simulink model "PMSM_2017b_1013"  (R2017b)
settings: Solver=FixedStepDiscrete  StartTime=0.0  StopTime=0.4  FixedStep=Ts  RelTol=1e-4  EnableMultiTasking=on
values from neighbouring files (symbols this model uses):
  AgSelector = 0    [initialization_1013.m]
  Ba = (Beta*J- Fl)/(1.5*P*flux)    [initialization_1013.m]
  Fl = 0.007*3/(100*pi)    (= 6.68450760986e-05)    [initialization_1013.m]
  flux = Kt/(1.5*P*sqrt(2))    [initialization_1013.m]
  fpwm = 1e4    (= 10000)    [initialization_1013.m]
  Imax = 6*sqrt(2)    [initialization_1013.m]
  J = 9.96e-5    (= 9.96e-05)    [initialization_1013.m]
  K1 = wn^2    (= 1000000)    [initialization_1013.m]
  K2 = 2*fei/wn    (= 0.003)    [initialization_1013.m]
  K_resolver = 1    [initialization_1013.m]
  Ki_Cctrl_d = Rs/(4*Tpwm)    (= 22125)    [initialization_1013.m]
  Ki_Cctrl_q = Rs/(4*Tpwm)    (= 22125)    [initialization_1013.m]
  Ki_Spdctrl = Beta*Kp_Spdctrl    [initialization_1013.m]
  Ki_Spdctrl_2 = 0.12*(pi*J)/(6000*P*flux*Tpwm^2)    [initialization_1013.m]
  Kp_Cctrl_d = Ld/(4*Tpwm)    (= 231.25)    [initialization_1013.m]
  Kp_Cctrl_q = Lq/(4*Tpwm)    (= 231.25)    [initialization_1013.m]
  Kp_Spdctrl = (Beta*J)/(1.5*P*flux)    [initialization_1013.m]
  Kp_Spdctrl_2 = 1*(pi*J)/(300*P*flux*Tpwm)    [initialization_1013.m]
  Kt = 1.32    [initialization_1013.m]
  Ld = Ls    (= 0.0925)    [initialization_1013.m]
  Lq = Ls    (= 0.0925)    [initialization_1013.m]
  Ls = 0.185/2    (= 0.0925)    [initialization_1013.m]
  P = 2    [initialization_1013.m]
  Rs = 17.7/2    (= 8.85)    [initialization_1013.m]
  SimMode = 1    [initialization_1013.m]
  TestCurrentController = 0    [initialization_1013.m]
  Tf = 0.08    [initialization_1013.m]
  Tpwm = 1e-4    (= 0.0001)    [initialization_1013.m]
  TqNorm = 0.6*9550/2500    (= 2.292)    [initialization_1013.m]
  Ts = 1e-6    (= 1e-06)    [initialization_1013.m]
  Udc = 230*sqrt(2)    [initialization_1013.m]
undefined symbols (not defined in the file or in its folder): A, B, DiscIntNeverNeededParam, f_LPF, f_LPF2, Init, K_SMO, Ki, Ki_PLL_SMO, Kp, Kp_PLL_SMO, LowerLimit, rate, UpperLimit
libraries: simulink x11, powerlib x7
(part 1 of 2)
settings Model: Creator=Joey Zhang  LastModifiedBy=Z0091619
settings SolverCC: ZeroCrossControl=DisableAll
settings DataIOCC: LimitDataPoints=on  SaveFormat=Array  SignalLoggingSaveFormat=ModelDataLogs
settings OptimizationCC: ExpressionDepthLimit=2147483647  InitFltsAndDblsToZero=on  LifeSpan=inf
settings DebuggingCC: UnderspecifiedInitializationDetection=Classic  MergeDetectMultiDrivingBlocksExec=none  SolverPrmCheckMsg=warning  FcnCallInpInsideContextMsg=warning  StateNameClashWarn=warning  SFUnexpectedBacktrackingDiag=warning  SFNoUnconditionalDefaultTransitionDiag=warning  SFExecutionAtInitializationDiag=none
settings HardwareCC: ProdBitPerPointer=32  ProdBitPerSizeT=32  ProdBitPerPtrDiffT=32  ProdLargestAtomicFloat=None  ProdIntDivRoundTo=Undefined  ProdEndianess=Unspecified  ProdWordSize=32  ProdHWDeviceType=32-bit Generic
settings ModelReferenceCC: PropagateSignalLabelsOutOfModel=off
settings CodeAppCC: StateflowObjectComments=on
settings GRTTargetCC: TargetLangStandard=C89/C90 (ANSI)  GeneratePreprocessorConditionals=Disable all  CombineOutputUpdateFcns=off  GRTInterface=on
settings ConfigComp: CovMetricSettings=dw  CovHtmlReporting=on  CovSaveCumulativeToWorkspaceVar=on  CovSaveSingleToWorkspaceVar=on  CovExternalEMLEnable=off
settings SimscapeCC: SimscapeNormalizeSystem=off

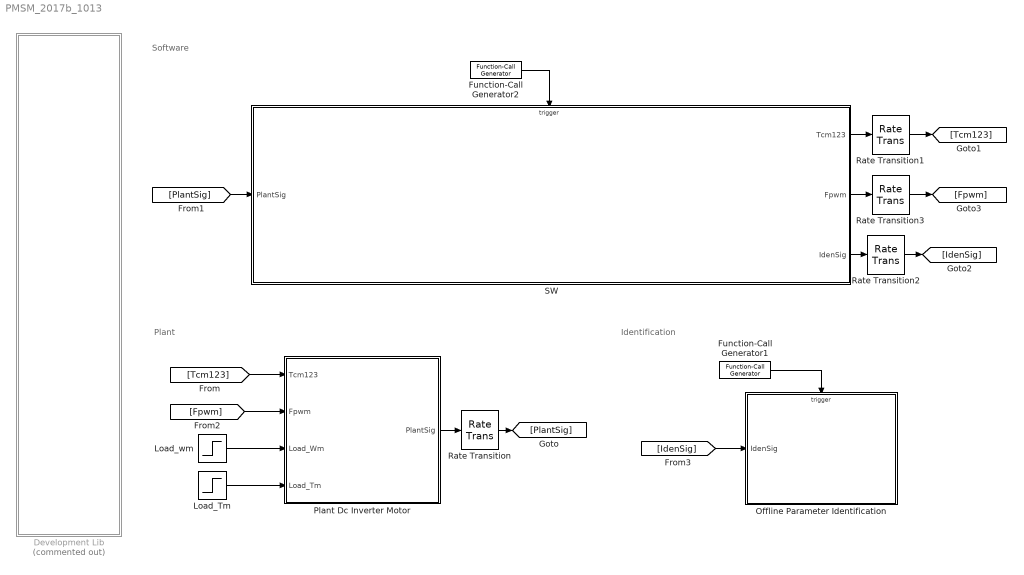
== system PMSM_2017b_1013 ==
  note: Software
  note: Plant
  note: Identification
  Development Lib : Subsystem  Commented=on
  Function-Call Generator1 : simulink/Ports & Subsystems/Function-Call Generator  sample_time=Tpwm  numberOfIterations=1
  Function-Call Generator2 : simulink/Ports & Subsystems/Function-Call Generator  sample_time=Tpwm  numberOfIterations=1
  Load_Tm : Step  After=TqNorm/2  SampleTime=0
  Load_wm : Step  Time=0.1  After=2500*pi/30  SampleTime=0
  Offline Parameter Identification : Subsystem
  Plant Dc Inverter Motor : Subsystem
  Rate Transition{,1..3} (4 alike) : RateTransition
  SW : Subsystem
  wires:
  Plant Dc Inverter Motor/1(PlantSig) -> Rate Transition/1
  SW/1(Tcm123) -> Rate Transition1/1
  SW/3(IdenSig) -> Rate Transition2/1
  [IdenSig] -> Offline Parameter Identification/1(IdenSig)
  Load_wm/1 -> Plant Dc Inverter Motor/3(Load_Wm)
  Load_Tm/1 -> Plant Dc Inverter Motor/4(Load_Tm)
  Function-Call Generator1/1 -> Offline Parameter Identification/Trigger
  Rate Transition/1 -> [PlantSig]
  [PlantSig] -> SW/1(PlantSig)
  [Tcm123] -> Plant Dc Inverter Motor/1(Tcm123)
  Rate Transition1/1 -> [Tcm123]
  Rate Transition2/1 -> [IdenSig]
  Function-Call Generator2/1 -> SW/Trigger
  SW/2(Fpwm) -> Rate Transition3/1
  Rate Transition3/1 -> [Fpwm]
  [Fpwm] -> Plant Dc Inverter Motor/2(Fpwm)

== system PMSM_2017b_1013/Development Lib ==
  AgRange(-pi,pi) : Subsystem
  Ag_atan2 : Subsystem
  Clamping_PI : Subsystem  Commented=on
  LPF1 : Subsystem
  Rate : Subsystem
  Speed : Subsystem  AncestorBlock=|  DialogController=POWERSYS.PowerSysDialog  mask(Discrete PI Controller){Kpw=Kp_Spdctrl, Kiw=Ki_Spdctrl, Ba=Ba, Par_Limits=[Imax -Imax], Init=0, Ts=-1}
      | powerlib_extras/Discrete 
      | Control Blocks/Discrete
      | PI Controller
      mask prompts: Kpw "Proportional gain (Kp):"; Kiw "Integral gain (Ki):"; Ba "feedback gain (Ba)"; Par_Limits "Output limits: [ Upper   Lower ]"; Init "Output initial value:"; Ts "Sample time:"
      mask help: This block implements a discrete PI controller.
      mask init:
      | UpperLimit=Par_Limits(1);
      | LowerLimit=Par_Limits(2);
      | power_initmask();
      mask Help: This block is part of a subset of blocks in the Extras library that does not have documentation associated with it, other than the block mask description.
      mask Display: disp('PI');
  TqEstimate : Subsystem  Commented=on
  UseMRASAg : Subsystem  Commented=on
  UseSMOAg : Subsystem  Commented=on
  pi-Id : Subsystem  AncestorBlock=|  DialogController=POWERSYS.PowerSysDialog  mask(Discrete PI Controller){Kp=Kp_Cctrl_d, Ki=Ki_Cctrl_d, Par_Limits=[Udc*sqrt(1/3) -Udc*sqrt(1/3)], Init=0, Ts=-1}
      | powerlib_extras/Discrete 
      | Control Blocks/Discrete
      | PI Controller
      mask prompts: Kp "Proportional gain (Kp):"; Ki "Integral gain (Ki):"; Par_Limits "Output limits: [ Upper   Lower ]"; Init "Output initial value:"; Ts "Sample time:"
      mask help: This block implements a discrete PI controller.
      mask init:
      | UpperLimit=Par_Limits(1);
      | LowerLimit=Par_Limits(2);
      | power_initmask();
      mask Help: This block is part of a subset of blocks in the Extras library that does not have documentation associated with it, other than the block mask description.
      mask Display: disp('PI');
  pi-Iq : Subsystem  AncestorBlock=|  DialogController=POWERSYS.PowerSysDialog  mask(Discrete PI Controller){Kp=Kp_Cctrl_q, Ki=Ki_Cctrl_q, Par_Limits=[Udc*sqrt(1/3) -Udc*sqrt(1/3)], Init=0, Ts=-1}
      | powerlib_extras/Discrete 
      | Control Blocks/Discrete
      | PI Controller
      mask prompts: Kp "Proportional gain (Kp):"; Ki "Integral gain (Ki):"; Par_Limits "Output limits: [ Upper   Lower ]"; Init "Output initial value:"; Ts "Sample time:"
      mask help: This block implements a discrete PI controller.
      mask init:
      | UpperLimit=Par_Limits(1);
      | LowerLimit=Par_Limits(2);
      | power_initmask();
      mask Help: This block is part of a subset of blocks in the Extras library that does not have documentation associated with it, other than the block mask description.
      mask Display: disp('PI');

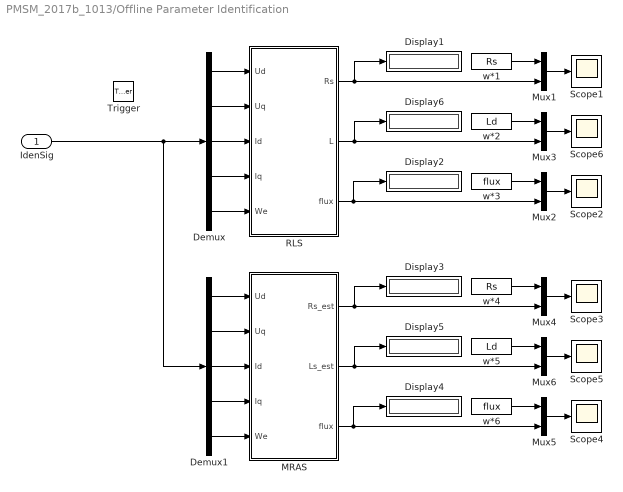
== system PMSM_2017b_1013/Offline Parameter Identification ==
  IdenSig : Inport
  Trigger : TriggerPort  TriggerType=function-call  VariantControl=Variant  PortDimensions=1
  Demux : Demux  Outputs=5
  Demux1 : Demux  Outputs=5
  Display{1..6} (6 alike) : Display
  MRAS : Subsystem
  Mux{1..6} (6 alike) : Mux  Inputs=2
  RLS : Subsystem
  Scope{1..6} (6 alike) : Scope
  w*1 : Constant  Value=Rs
  w*2 : Constant  Value=Ld
  w*3 : Constant  Value=flux
  w*4 : Constant  Value=Rs
  w*5 : Constant  Value=Ld
  w*6 : Constant  Value=flux
  wires:
  Mux3/1 -> Scope6/1
  RLS/2(L) -> Display6/1, Mux3/2
  w*2/1 -> Mux3/1
  w*1/1 -> Mux1/1
  RLS/1(Rs) -> Mux1/2, Display1/1
  Mux1/1 -> Scope1/1
  Mux2/1 -> Scope2/1
  RLS/3(flux) -> Display2/1, Mux2/2
  w*3/1 -> Mux2/1
  Demux/1 -> RLS/1(Ud)
  Demux/2 -> RLS/2(Uq)
  Demux/3 -> RLS/3(Id)
  Demux/4 -> RLS/4(Iq)
  Demux/5 -> RLS/5(We)
  Demux1/5 -> MRAS/5(We)
  Demux1/4 -> MRAS/4(Iq)
  Demux1/3 -> MRAS/3(Id)
  Demux1/2 -> MRAS/2(Uq)
  Demux1/1 -> MRAS/1(Ud)
  IdenSig/1 -> Demux1/1, Demux/1
  w*6/1 -> Mux5/1
  MRAS/3(flux) -> Mux5/2, Display4/1
  Mux5/1 -> Scope4/1
  Mux4/1 -> Scope3/1
  MRAS/1(Rs_est) -> Display3/1, Mux4/2
  w*4/1 -> Mux4/1
  w*5/1 -> Mux6/1
  MRAS/2(Ls_est) -> Mux6/2, Display5/1
  Mux6/1 -> Scope5/1

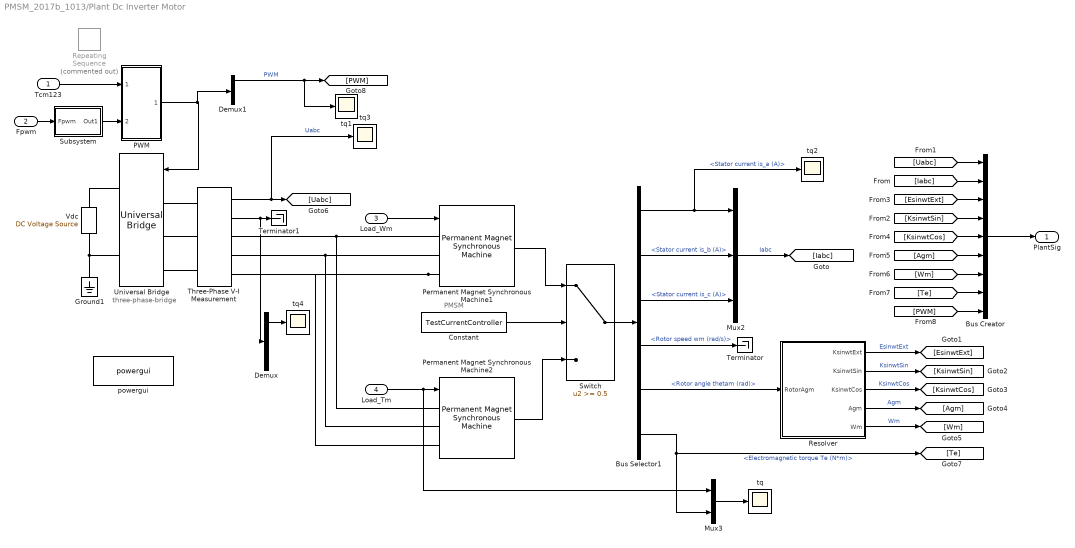
== system PMSM_2017b_1013/Plant Dc Inverter Motor ==
  note: three-phase-bridge
  note: PMSM
  Tcm123 : Inport
  Fpwm : Inport  Port=2
  Load_Wm : Inport  Port=3
  Load_Tm : Inport  Port=4
  Bus Creator : BusCreator  Inputs=9
  Bus Selector1 : BusSelector  OutputSignals=Stator current is_a (A),Stator current is_b (A),Stator current is_c (A),Rotor speed wm (rad/s),Rotor angle thetam (rad),Electromagnetic torque Te (N*m)
  Constant : Constant  Value=TestCurrentController
  Demux : Demux  Outputs=3
  Demux1 : Demux  Outputs=6
  Ground1 : powerlib/Elements/Ground  LConnTagsString=a
  Mux2 : Mux  Inputs=3
  Mux3 : Mux  Inputs=2
  PWM : Subsystem
  Permanent Magnet Synchronous Machine1 : powerlib/Machines/Permanent Magnet Synchronous Machine  NbPhases=3  FluxDistribution=Sinusoidal  RotorType=Round  MechanicalLoad=Speed w  PresetModel=No  ShowDetailedParameters=on  MeasurementBus=off  Resistance=Rs  Inductance=8.5e-3  dqInductances=[Ld Lq]  La=Ls  MachineConstant=Flux linkage established by magnets (V.s)  Flux=flux  VoltageCst=112.8644  TorqueCst=0.93338  Flat=120  Mechanical=[J Fl P Tf]  PolePairs=P  InitialConditions=[0,0,0,0]  InitialConditions5ph=[0 0 0 0 0 0]  TsPowergui=0  TsBlock=-1  RefAngle=Aligned with phase A axis (original Park)
      settings: SourceProductName=Simscape Power Systems
  Permanent Magnet Synchronous Machine2 : powerlib/Machines/Permanent Magnet Synchronous Machine  NbPhases=3  FluxDistribution=Sinusoidal  RotorType=Salient-pole  MechanicalLoad=Torque Tm  PresetModel=No  ShowDetailedParameters=on  MeasurementBus=off  Resistance=Rs  Inductance=8.5e-3  dqInductances=[Ld Lq]  La=Ls  MachineConstant=Flux linkage established by magnets (V.s)  Flux=flux  VoltageCst=112.8644  TorqueCst=0.93338  Flat=120  Mechanical=[J Fl P Tf]  PolePairs=P  InitialConditions=[0,0,0,0]  InitialConditions5ph=[0 0 0 0 0 0]  TsPowergui=0  TsBlock=-1  RefAngle=Aligned with phase A axis (original Park)
      settings: SourceProductName=Simscape Power Systems
  Repeating Sequence : simulink/Sources/Repeating Sequence  Commented=on  rep_seq_t=[0 Tpwm/2 Tpwm]  rep_seq_y=[0 Tpwm/2 0]
  Resolver : Subsystem
  Subsystem : Subsystem
  Switch : Switch  Threshold=0.5
  Terminator : Terminator
  Terminator1 : Terminator
  Three-Phase V-I Measurement : powerlib/Measurements/Three-Phase V-I Measurement  VoltageMeasurement=phase-to-ground  SetLabelV=off  LabelV=Vabc  Vpu=off  VpuLL=off  CurrentMeasurement=yes  SetLabelI=off  LabelI=Iabc  Ipu=off  Pbase=100e6  Vbase=500e3  OutputType=Complex  PhasorSimulation=off  PSBequivalent=0
  Universal Bridge : powerlib/Power Electronics/Universal Bridge  Arms=3  SnubberResistance=1e5  SnubberCapacitance=inf  Device=MOSFET / Diodes  Ron=1e-3  Lon=0  ForwardVoltages="[  0  0  ]"  ForwardVoltage=0  GTOparameters=[ 10e-6 , 20e-6 ]  IGBTparameters=[ 1e-6 , 2e-6 ]  Measurements=All voltages and currents  Measurements_2=None  converterType=Rectifier
  Vdc : powerlib/Electrical Sources/DC Voltage Source  Amplitude=Udc  Measurements=Voltage
  powergui : powerlib/powergui  SimulationMode=Discrete  SampleTime=Ts  frequency=60  Iterations=50  frequencyindice=0  Pbase=100e6  ErrMax=1e-4  UnitsV=kV  UnitsW=MW  buscounter=0  FunctionMessages=off  echomessages=off  EnableUseOfTLC=off  CurrentSourceSwitches=off  DisableSnubberDevices=off  DisableRonSwitches=off  DisableVfSwitches=off  DisplayEquations=off  SolverType=Backward Euler  Interpol=off  ExternalGateDelay=off  methode=off  Ts=0  x0status=blocks  SPID=off  SwTol=0  HookPort=off  RestoreLinks=warning  ResistiveCurrentMeasurement=off  Frange=[0:2:500]  Ylog=off  Xlog=on  ShowGrid=off  save=off  variable=ZData  structure=simout  ZoomFFT=off  StartTime=0.0  cycles=3  DisplayStyle=1  fundamental=60  FreqAxis=off  MaxFrequency=1000  frequencyindicesteady=1  RmsSteady=1  display=off
  tq{,1..4} (5 alike) : Scope
  PlantSig : Outport
  wires:
  Permanent Magnet Synchronous Machine1/1 -> Switch/1
  Switch/1 -> Bus Selector1/1
  Constant/1 -> Switch/2
  Mux3/1 -> tq/1
  Tcm123/1 -> PWM/1(Tcm123)
  Three-Phase V-I Measurement/1 -> tq3/1, [Uabc]  "Uabc"
  Mux2/1 -> [Iabc]  "Iabc"
  Permanent Magnet Synchronous Machine2/1 -> Switch/3
  Load_Tm/1 -> Mux3/1, Permanent Magnet Synchronous Machine2/1
  Bus Selector1/1 -> tq2/1, Mux2/1  "<Stator current is_a (A)>"
  Bus Selector1/2 -> Mux2/2  "<Stator current is_b (A)>"
  Bus Selector1/3 -> Mux2/3  "<Stator current is_c (A)>"
  Bus Selector1/5 -> Resolver/1(RotorAgm)  "<Rotor angle thetam (rad)>"
  Bus Selector1/4 -> Terminator/1  "<Rotor speed wm (rad/s)>"
  Three-Phase V-I Measurement/2 -> Demux/1, Terminator1/1
  Resolver/1(KsinwtExt) -> [EsinwtExt]  "EsinwtExt"
  Resolver/2(KsinwtSin) -> [KsinwtSin]  "KsinwtSin"
  Resolver/3(KsinwtCos) -> [KsinwtCos]  "KsinwtCos"
  Resolver/4(Agm) -> [Agm]  "Agm"
  Resolver/5(Wm) -> [Wm]  "Wm"
  Bus Selector1/6 -> [Te], Mux3/2  "<Electromagnetic torque Te (N*m)>"
  Bus Creator/1 -> PlantSig/1
  [Uabc] -> Bus Creator/1
  [Iabc] -> Bus Creator/2
  [EsinwtExt] -> Bus Creator/3
  [KsinwtSin] -> Bus Creator/4
  [KsinwtCos] -> Bus Creator/5
  [Agm] -> Bus Creator/6
  [Wm] -> Bus Creator/7
  [Te] -> Bus Creator/8
  Demux/1 -> tq4/1
  Load_Wm/1 -> Permanent Magnet Synchronous Machine1/1
  PWM/1(PWM) -> Demux1/1, Universal Bridge/1
  Demux1/1 -> tq1/1, [PWM]  "PWM"
  [PWM] -> Bus Creator/9
  Fpwm/1 -> Subsystem/1(Fpwm)
  Subsystem/1(Out1) -> PWM/2(Carrier)
  connections:
  Universal Bridge/RConn1 -- Vdc/RConn1
  Universal Bridge/RConn2 -- Ground1/LConn1 -- Vdc/LConn1
  Permanent Magnet Synchronous Machine1/LConn1 -- Three-Phase V-I Measurement/RConn1 -- Permanent Magnet Synchronous Machine2/LConn1
  Permanent Magnet Synchronous Machine1/LConn2 -- Three-Phase V-I Measurement/RConn2 -- Permanent Magnet Synchronous Machine2/LConn2
  Permanent Magnet Synchronous Machine1/LConn3 -- Permanent Magnet Synchronous Machine2/LConn3 -- Three-Phase V-I Measurement/RConn3
  Three-Phase V-I Measurement/LConn3 -- Universal Bridge/LConn3
  Universal Bridge/LConn2 -- Three-Phase V-I Measurement/LConn2
  Universal Bridge/LConn1 -- Three-Phase V-I Measurement/LConn1

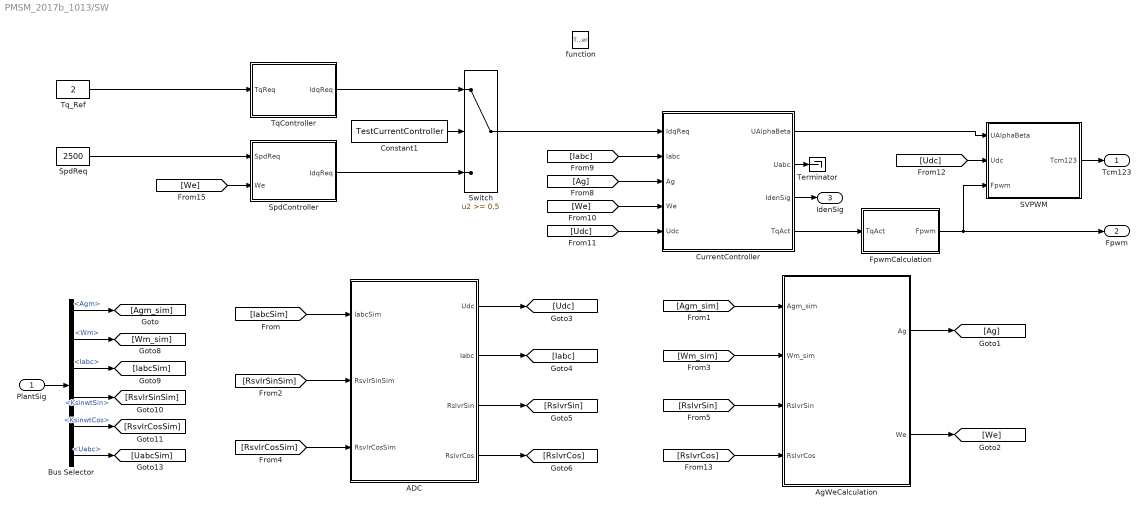
== system PMSM_2017b_1013/SW ==
  PlantSig : Inport
  function : TriggerPort  TriggerType=function-call  VariantControl=Variant
  ADC : Subsystem
  AgWeCalculation : Subsystem
  Bus Selector : BusSelector  OutputSignals=Agm,Wm,Iabc,KsinwtSin,KsinwtCos,Uabc
  Constant1 : Constant  Value=TestCurrentController
  CurrentController : Subsystem
  FpwmCalculation : Subsystem
  SVPWM : Subsystem
  SpdController : Subsystem
  SpdReq : Constant  Value=2500
  Switch : Switch  Threshold=0.5
  Terminator : Terminator
  TqController : Subsystem
  Tq_Ref : Constant  Value=2
  Tcm123 : Outport
  Fpwm : Outport  Port=2
  IdenSig : Outport  Port=3
  wires:
  Constant1/1 -> Switch/2
  SVPWM/1(Tcm123) -> Tcm123/1
  Tq_Ref/1 -> TqController/1(TqReq)
  TqController/1(IdqReq) -> Switch/1
  SpdReq/1 -> SpdController/1(SpdReq)
  SpdController/1(IdqReq) -> Switch/3
  Switch/1 -> CurrentController/1(IdqReq)
  CurrentController/1(UAlphaBeta) -> SVPWM/1(UAlphaBeta)
  AgWeCalculation/1(Ag) -> [Ag]
  AgWeCalculation/2(We) -> [We]
  [Ag] -> CurrentController/3(Ag)
  [Iabc] -> CurrentController/2(Iabc)
  [We] -> CurrentController/4(We)
  [Udc] -> CurrentController/5(Udc)
  [Udc] -> SVPWM/2(Udc)
  ADC/1(Udc) -> [Udc]
  ADC/2(Iabc) -> [Iabc]
  ADC/4(RslvrCos) -> [RslvrCos]
  ADC/3(RslvrSin) -> [RslvrSin]
  [Agm_sim] -> AgWeCalculation/1(Agm_sim)
  [Wm_sim] -> AgWeCalculation/2(Wm_sim)
  [RslvrSin] -> AgWeCalculation/3(RslvrSin)
  [RslvrCos] -> AgWeCalculation/4(RslvrCos)
  [We] -> SpdController/2(We)
  CurrentController/2(Uabc) -> Terminator/1
  PlantSig/1 -> Bus Selector/1
  Bus Selector/1 -> [Agm_sim]  "<Agm>"
  Bus Selector/2 -> [Wm_sim]  "<Wm>"
  Bus Selector/3 -> [IabcSim]  "<Iabc>"
  Bus Selector/4 -> [RsvlrSinSim]  "<KsinwtSin>"
  Bus Selector/5 -> [RsvlrCosSim]  "<KsinwtCos>"
  [IabcSim] -> ADC/1(IabcSim)
  [RsvlrCosSim] -> ADC/3(RsvlrCosSim)
  [RsvlrSinSim] -> ADC/2(RsvlrSinSim)
  Bus Selector/6 -> [UabcSim]  "<Uabc>"
  CurrentController/3(IdenSig) -> IdenSig/1
  CurrentController/4(TqAct) -> FpwmCalculation/1(TqAct)
  FpwmCalculation/1(Fpwm) -> Fpwm/1, SVPWM/3(Fpwm)

== system PMSM_2017b_1013/Development Lib/AgRange(-pi,pi) ==
  note: To make the Ag is in the range of [-pi,pi]
  Ag_RangeInf : Inport
  Constant : Constant  Value=pi
  Constant2 : Constant  Value=2*pi
  Mod : Math  Operator=mod  SaturateOnIntegerOverflow=on
  Relational Operator : RelationalOperator  OutDataTypeStr=boolean  RndMeth=Simplest
  Sum : Sum  Inputs=|+-
  Switch2 : Switch  Criteria=u2 > Threshold  Threshold=0.5
  Ag : Outport
  wires:
  Sum/1 -> Switch2/1
  Relational Operator/1 -> Switch2/2
  Ag_RangeInf/1 -> Mod/1
  Constant/1 -> Relational Operator/2
  Constant2/1 -> Sum/2, Mod/2
  Mod/1 -> Sum/1, Switch2/3, Relational Operator/1
  Switch2/1 -> Ag/1

== system PMSM_2017b_1013/Development Lib/Ag_atan2 ==
  Sin : Inport
  cos : Inport  Port=2
  Discrete Derivative : simulink/Discrete/Discrete Derivative  gainval=1.0  ICPrevScaledInput=0.0  OutMin=[]  OutMax=[]  OutDataType=fixdt(1, 16)  OutScaling=2^-10  DoSatur=off
  Sin1 : Trigonometry  Operator=atan2
  Ag : Outport
  we : Outport  Port=2
  wires:
  Sin/1 -> Sin1/1
  Sin1/1 -> Ag/1, Discrete Derivative/1
  Discrete Derivative/1 -> we/1
  cos/1 -> Sin1/2

== system PMSM_2017b_1013/Development Lib/Clamping_PI ==
  Error : Inport
  Udc : Inport  Port=2
  Abs : Abs
  Constant : Constant
  Constant1 : Constant  Value=0
  Discrete-Time Integrator : DiscreteIntegrator  IntegratorMethod=Integration: Trapezoidal  InitialCondition=Init  SampleTime=-1  UpperSaturationLimit=UpperLimit  LowerSaturationLimit=LowerLimit  ICPrevOutput=DiscIntNeverNeededParam  ICPrevScaledInput=DiscIntNeverNeededParam
  Gain : Gain  Gain=1/sqrt(3)
  Gain1 : Gain  Gain=-1
  Kp4 : Gain  Gain=Kp  SaturateOnIntegerOverflow=on  OutDataTypeStr=Inherit: Same as input  ParamDataTypeStr=Inherit: Same as input
  Kp5 : Gain  Gain=Ki  SaturateOnIntegerOverflow=on  OutDataTypeStr=Inherit: Same as input  ParamDataTypeStr=Inherit: Same as input
  Product : Product
  Relational Operator : RelationalOperator  OutDataTypeStr=boolean  RndMeth=Simplest
  Saturation Dynamic : simulink/Discontinuities/Saturation Dynamic  OutMin=[]  OutMax=[]  OutDataTypeStr=Inherit: Same as second input  OutDataType=fixdt(1, 16)  OutScaling=2^-10  DoSatur=off
  Sum6 : Sum  InputSameDT=on  OutDataTypeStr=Inherit: Same as first input
  Switch : Switch  Criteria=u2 > Threshold  Threshold=0.5
  Zero-Order Hold : ZeroOrderHold  SampleTime=-1
  Out : Outport  InitialOutput=0
  wires:
  Zero-Order Hold/1 -> Sum6/1
  Error/1 -> Kp5/1, Kp4/1
  Kp4/1 -> Zero-Order Hold/1
  Sum6/1 -> Saturation Dynamic/2, Abs/1
  Discrete-Time Integrator/1 -> Sum6/2
  Udc/1 -> Gain/1
  Gain/1 -> Saturation Dynamic/1, Relational Operator/1, Gain1/1
  Saturation Dynamic/1 -> Out/1
  Relational Operator/1 -> Switch/2
  Constant1/1 -> Switch/3
  Constant/1 -> Switch/1
  Switch/1 -> Product/2
  Kp5/1 -> Product/1
  Product/1 -> Discrete-Time Integrator/1
  Gain1/1 -> Saturation Dynamic/3
  Abs/1 -> Relational Operator/2

== system PMSM_2017b_1013/Development Lib/LPF1 ==
  u_in : Inport
  Add : Sum  Inputs=+-
  Add1 : Sum
  Constant : Constant  Value=Ts
  Constant1 : Constant  Value=f_LPF2
  Gain3 : Gain  Gain=2*pi
  Product : Product
  Product1 : Product
  Unit Delay : UnitDelay  SampleTime=-1
  u_out : Outport
  wires:
  Add1/1 -> Unit Delay/1, u_out/1
  Product/1 -> Product1/1
  Add/1 -> Product1/2
  Product1/1 -> Add1/1
  Gain3/1 -> Product/2
  Constant/1 -> Product/1
  Constant1/1 -> Gain3/1
  u_in/1 -> Add/1
  Unit Delay/1 -> Add/2, Add1/2

== system PMSM_2017b_1013/Development Lib/Rate ==
  In : Inport
  Abs : Abs
  Add : Sum  Inputs=+-
  Add1 : Sum
  Constant : Constant  Value=rate
  Product : Product
  Relational Operator : RelationalOperator  Operator=>  OutDataTypeStr=boolean  RndMeth=Simplest
  Switch1 : Switch  Criteria=u2 > Threshold
  Unit Delay : UnitDelay  SampleTime=-1
  Out1 : Outport
  wires:
  Relational Operator/1 -> Switch1/2
  Switch1/1 -> Out1/1
  In/1 -> Add1/1, Product/1, Switch1/3, Abs/1
  Unit Delay/1 -> Add/2
  Add/1 -> Relational Operator/1
  Constant/1 -> Product/2, Relational Operator/2
  Abs/1 -> Unit Delay/1, Add/1
  Add1/1 -> Switch1/1
  Product/1 -> Add1/2

== system PMSM_2017b_1013/Development Lib/Speed ==
  note: Discrete PID Controller
  Error : Inport
  Discrete-Time Integrator : DiscreteIntegrator  IntegratorMethod=Integration: Trapezoidal  InitialCondition=Init  SampleTime=-1  LimitOutput=on  UpperSaturationLimit=UpperLimit  LowerSaturationLimit=LowerLimit  ICPrevOutput=DiscIntNeverNeededParam  ICPrevScaledInput=DiscIntNeverNeededParam
  Kp1 : Gain  Gain=Ba  SaturateOnIntegerOverflow=on  OutDataTypeStr=Inherit: Same as input  ParamDataTypeStr=Inherit: Same as input
  Kp4 : Gain  Gain=Kpw  SaturateOnIntegerOverflow=on  OutDataTypeStr=Inherit: Same as input  ParamDataTypeStr=Inherit: Same as input
  Kp5 : Gain  Gain=Kiw  SaturateOnIntegerOverflow=on  OutDataTypeStr=Inherit: Same as input  ParamDataTypeStr=Inherit: Same as input
  Saturation2 : Saturate  UpperLimit=UpperLimit  LowerLimit=LowerLimit
  Scope : Scope
  Sum6 : Sum  Inputs=++-  SaturateOnIntegerOverflow=on  InputSameDT=on  OutDataTypeStr=Inherit: Same as first input
  Zero-Order Hold : ZeroOrderHold  SampleTime=-1
  Out : Outport  InitialOutput=0
  wires:
  Error/1 -> Kp4/1, Kp5/1
  Zero-Order Hold/1 -> Scope/1, Sum6/1
  Saturation2/1 -> Out/1
  Discrete-Time Integrator/1 -> Sum6/2
  Kp4/1 -> Zero-Order Hold/1
  Sum6/1 -> Saturation2/1
  Kp1/1 -> Sum6/3
  [Nr] -> Kp1/1
  Kp5/1 -> Discrete-Time Integrator/1

== system PMSM_2017b_1013/Development Lib/TqEstimate ==
  iq : Inport
  Gain : Gain  Gain=1.5*P*flux
  TqEst : Outport
  wires:
  Gain/1 -> TqEst/1
  iq/1 -> Gain/1

== system PMSM_2017b_1013/Development Lib/UseMRASAg ==
  note: 采用模型参考自适应算法估算电角度
  ud : Inport
  uq : Inport  Port=2
  id : Inport  Port=3
  iq : Inport  Port=4
  MRAS : Subsystem
  Ag_SMO : Outport
  We_SMO : Outport  Port=2

== system PMSM_2017b_1013/Development Lib/UseSMOAg ==
  note: 采用滑模控制 进行角度估算
  Uabc : Inport
  Iabc : Inport  Port=2
  Atan : Subsystem
  "PLL " : Subsystem
  Scope : Scope  NumInputPorts=2
  Scope1 : Scope  NumInputPorts=2
  Subsystem : Subsystem
  Ag_SMO : Outport
  We_SMO : Outport  Port=2
  wires:
  Iabc/1 -> Subsystem/2(Iabc)
  Uabc/1 -> Subsystem/1(Uabc)
  Subsystem/1(E_AlphaBeta) -> Atan/1(E_AlphaBeta), "PLL "/1(E_AlphaBeta)
  Atan/1(Ag_SMO) -> Scope/1
  Atan/2(we_SMO) -> Scope/2
  "PLL "/1(Ag_SMO) -> Ag_SMO/1, Scope1/1
  "PLL "/2(we_SMO) -> We_SMO/1, Scope1/2

== system PMSM_2017b_1013/Development Lib/pi-Id ==
  note: Discrete PID Controller
  Error : Inport  SampleTime=Ts
  Discrete-Time Integrator : DiscreteIntegrator  IntegratorMethod=Integration: Trapezoidal  InitialCondition=Init  SampleTime=-1  LimitOutput=on  UpperSaturationLimit=UpperLimit  LowerSaturationLimit=LowerLimit  ICPrevOutput=DiscIntNeverNeededParam  ICPrevScaledInput=DiscIntNeverNeededParam
  Kp4 : Gain  Gain=Kp  SaturateOnIntegerOverflow=on  OutDataTypeStr=Inherit: Same as input  ParamDataTypeStr=Inherit: Same as input
  Kp5 : Gain  Gain=Ki  SaturateOnIntegerOverflow=on  OutDataTypeStr=Inherit: Same as input  ParamDataTypeStr=Inherit: Same as input
  Saturation2 : Saturate  UpperLimit=UpperLimit  LowerLimit=LowerLimit
  Sum6 : Sum  SaturateOnIntegerOverflow=on  InputSameDT=on  OutDataTypeStr=Inherit: Same as first input
  Zero-Order Hold : ZeroOrderHold  SampleTime=-1
  Out : Outport  SampleTime=Ts  InitialOutput=0
  wires:
  Zero-Order Hold/1 -> Sum6/1
  Saturation2/1 -> Out/1
  Discrete-Time Integrator/1 -> Sum6/2
  Kp4/1 -> Zero-Order Hold/1
  Sum6/1 -> Saturation2/1
  Error/1 -> Kp5/1, Kp4/1
  Kp5/1 -> Discrete-Time Integrator/1

== system PMSM_2017b_1013/Development Lib/pi-Iq ==
  note: Discrete PID Controller
  Error : Inport  SampleTime=Ts
  Discrete-Time Integrator : DiscreteIntegrator  IntegratorMethod=Integration: Trapezoidal  InitialCondition=Init  SampleTime=-1  LimitOutput=on  UpperSaturationLimit=UpperLimit  LowerSaturationLimit=LowerLimit  ICPrevOutput=DiscIntNeverNeededParam  ICPrevScaledInput=DiscIntNeverNeededParam
  Kp4 : Gain  Gain=Kp  SaturateOnIntegerOverflow=on  OutDataTypeStr=Inherit: Same as input  ParamDataTypeStr=Inherit: Same as input
  Kp5 : Gain  Gain=Ki  SaturateOnIntegerOverflow=on  OutDataTypeStr=Inherit: Same as input  ParamDataTypeStr=Inherit: Same as input
  Saturation2 : Saturate  UpperLimit=UpperLimit  LowerLimit=LowerLimit
  Sum6 : Sum  SaturateOnIntegerOverflow=on  InputSameDT=on  OutDataTypeStr=Inherit: Same as first input
  Zero-Order Hold : ZeroOrderHold  SampleTime=-1
  Out : Outport  SampleTime=Ts  InitialOutput=0
  wires:
  Zero-Order Hold/1 -> Sum6/1
  Saturation2/1 -> Out/1
  Discrete-Time Integrator/1 -> Sum6/2
  Kp4/1 -> Zero-Order Hold/1
  Sum6/1 -> Saturation2/1
  Error/1 -> Kp5/1, Kp4/1
  Kp5/1 -> Discrete-Time Integrator/1

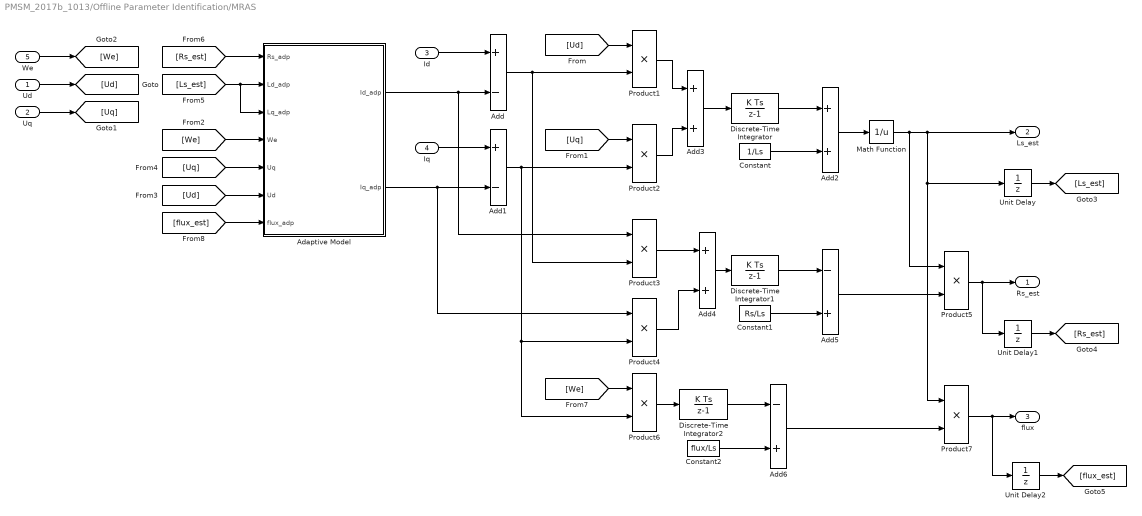
== system PMSM_2017b_1013/Offline Parameter Identification/MRAS ==
  Ud : Inport
  Uq : Inport  Port=2
  Id : Inport  Port=3
  Iq : Inport  Port=4
  We : Inport  Port=5
  Adaptive Model : Subsystem
  Add : Sum  Inputs=+-
  Add1 : Sum  Inputs=+-
  Add2 : Sum
  Add3 : Sum
  Add4 : Sum
  Add5 : Sum  Inputs=-+
  Add6 : Sum  Inputs=-+
  Constant : Constant  Value=1/Ls
  Constant1 : Constant  Value=Rs/Ls
  Constant2 : Constant  Value=flux/Ls
  Discrete-Time Integrator : DiscreteIntegrator  SampleTime=-1  UpperSaturationLimit=UpperLimit  LowerSaturationLimit=LowerLimit  ICPrevOutput=DiscIntNeverNeededParam  ICPrevScaledInput=DiscIntNeverNeededParam
  Discrete-Time Integrator1 : DiscreteIntegrator  SampleTime=-1  UpperSaturationLimit=UpperLimit  LowerSaturationLimit=LowerLimit  ICPrevOutput=DiscIntNeverNeededParam  ICPrevScaledInput=DiscIntNeverNeededParam
  Discrete-Time Integrator2 : DiscreteIntegrator  SampleTime=-1  UpperSaturationLimit=UpperLimit  LowerSaturationLimit=LowerLimit  ICPrevOutput=DiscIntNeverNeededParam  ICPrevScaledInput=DiscIntNeverNeededParam
  Math Function : Math  Operator=reciprocal  SaturateOnIntegerOverflow=on
  Product{1..7} (7 alike) : Product
  Unit Delay : UnitDelay  InitialCondition=Ls  SampleTime=-1
  Unit Delay1 : UnitDelay  InitialCondition=Rs  SampleTime=-1
  Unit Delay2 : UnitDelay  InitialCondition=flux  SampleTime=-1
  Rs_est : Outport
  Ls_est : Outport  Port=2
  flux : Outport  Port=3
  wires:
  Id/1 -> Add/1
  Iq/1 -> Add1/1
  Adaptive Model/2(Iq_adp) -> Product4/1, Add1/2
  Discrete-Time Integrator/1 -> Add2/1
  Ud/1 -> [Ud]
  [Ud] -> Product1/1
  We/1 -> [We]
  [Uq] -> Product2/1
  Add1/1 -> Product6/2, Product4/2, Product2/2
  Uq/1 -> [Uq]
  Product1/1 -> Add3/1
  Product2/1 -> Add3/2
  Add3/1 -> Discrete-Time Integrator/1
  Add2/1 -> Math Function/1
  Math Function/1 -> Product5/1, Product7/1, Unit Delay/1, Ls_est/1
  Constant/1 -> Add2/2
  [We] -> Adaptive Model/4(We)
  [Ud] -> Adaptive Model/6(Ud)
  [Uq] -> Adaptive Model/5(Uq)
  Adaptive Model/1(Id_adp) -> Product3/1, Add/2
  Add/1 -> Product3/2, Product1/2
  Product3/1 -> Add4/1
  Product4/1 -> Add4/2
  Constant1/1 -> Add5/2
  Discrete-Time Integrator1/1 -> Add5/1
  Add4/1 -> Discrete-Time Integrator1/1
  Add5/1 -> Product5/2
  Product5/1 -> Unit Delay1/1, Rs_est/1
  Unit Delay/1 -> [Ls_est]
  [Ls_est] -> Adaptive Model/3(Lq_adp), Adaptive Model/2(Ld_adp)
  Unit Delay1/1 -> [Rs_est]
  [Rs_est] -> Adaptive Model/1(Rs_adp)
  [We] -> Product6/1
  Product6/1 -> Discrete-Time Integrator2/1
  Constant2/1 -> Add6/2
  Discrete-Time Integrator2/1 -> Add6/1
  Add6/1 -> Product7/2
  Product7/1 -> Unit Delay2/1, flux/1
  Unit Delay2/1 -> [flux_est]
  [flux_est] -> Adaptive Model/7(flux_adp)

== system PMSM_2017b_1013/Offline Parameter Identification/RLS ==
  Ud : Inport
  Uq : Inport  Port=2
  Id : Inport  Port=3
  Iq : Inport  Port=4
  We : Inport  Port=5
  RLS : Subsystem
  RSL_1 : Subsystem
  Rs : Outport
  L : Outport  Port=2
  flux : Outport  Port=3
  wires:
  Ud/1 -> RLS/1(Ud), RSL_1/1(Ud)
  Uq/1 -> RLS/2(Uq), RSL_1/2(Uq)
  Iq/1 -> RLS/4(Iq), RSL_1/4(Iq)
  We/1 -> RLS/5(We), RSL_1/5(We)
  RSL_1/1(Rs) -> Rs/1
  RSL_1/2(L) -> L/1
  RSL_1/3(flux) -> flux/1
  Id/1 -> RLS/3(Id), RSL_1/3(Id)

== system PMSM_2017b_1013/Plant Dc Inverter Motor/PWM ==
  Tcm123 : Inport
  Carrier : Inport  Port=2
  Add : Sum  Inputs=+-
  Add1 : Sum  Inputs=+-
  Add2 : Sum  Inputs=+-
  Data Type Conversion : DataTypeConversion  OutDataTypeStr=double
  Data Type Conversion1 : DataTypeConversion  OutDataTypeStr=double
  Data Type Conversion2 : DataTypeConversion  OutDataTypeStr=double
  Demux : Demux  Outputs=3
  Logical Operator : Logic  Operator=NOT  AllPortsSameDT=off  OutDataTypeStr=boolean
  Logical Operator1 : Logic  Operator=NOT  AllPortsSameDT=off  OutDataTypeStr=boolean
  Logical Operator2 : Logic  Operator=NOT  AllPortsSameDT=off  OutDataTypeStr=boolean
  Mux : Mux  Inputs=6
  Mux1 : Mux  Inputs=2
  Relay : Relay  OffSwitchValue=-eps
  Relay1 : Relay  OffSwitchValue=-eps
  Relay2 : Relay  OffSwitchValue=-eps
  Te1 : Scope
  Te4 : Scope
  PWM : Outport
  wires:
  Demux/3 -> Add2/2
  Demux/2 -> Add1/2
  Demux/1 -> Te1/1, Mux1/2, Add/2
  Relay/1 -> Mux/5, Logical Operator2/1
  Relay1/1 -> Mux/3, Logical Operator1/1
  Mux/1 -> PWM/1
  Data Type Conversion/1 -> Mux/2
  Data Type Conversion1/1 -> Mux/4
  Data Type Conversion2/1 -> Mux/6
  Logical Operator2/1 -> Data Type Conversion2/1
  Logical Operator1/1 -> Data Type Conversion1/1
  Logical Operator/1 -> Data Type Conversion/1
  Add1/1 -> Relay1/1
  Add2/1 -> Relay/1
  Add/1 -> Relay2/1
  Tcm123/1 -> Demux/1
  Mux1/1 -> Te4/1
  Relay2/1 -> Mux/1, Logical Operator/1
  Carrier/1 -> Mux1/1, Add/1, Add2/1, Add1/1

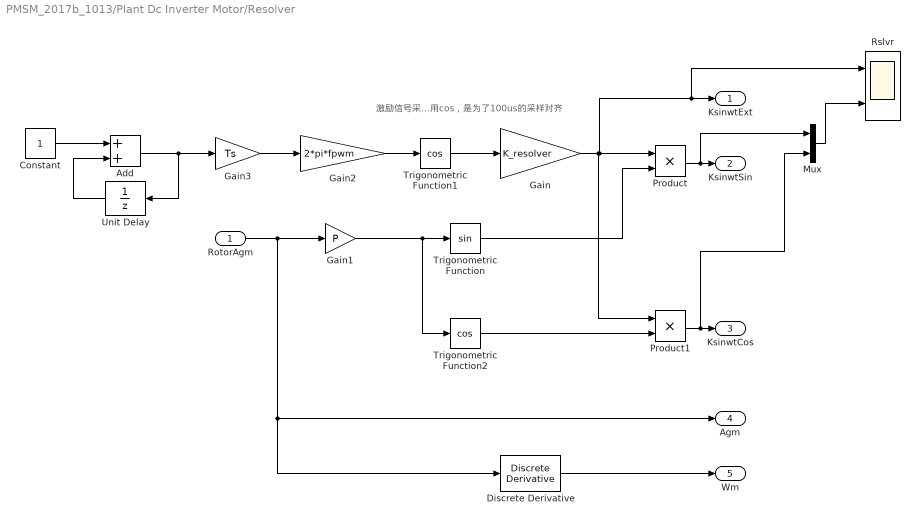
== system PMSM_2017b_1013/Plant Dc Inverter Motor/Resolver ==
  note: 激励信号采用cos，是为了100us的采样对齐
  RotorAgm : Inport
  Add : Sum
  Constant : Constant
  Discrete Derivative : simulink/Discrete/Discrete Derivative  gainval=1.0  ICPrevScaledInput=0.0  OutMin=[]  OutMax=[]  OutDataType=fixdt(1, 16)  OutScaling=2^-10  DoSatur=off
  Gain : Gain  Gain=K_resolver
  Gain1 : Gain  Gain=P
  Gain2 : Gain  Gain=2*pi*fpwm
  Gain3 : Gain  Gain=Ts
  Mux : Mux  Inputs=2
  Product : Product
  Product1 : Product
  Rslvr : Scope  NumInputPorts=2
  Trigonometric Function : Trigonometry
  Trigonometric Function1 : Trigonometry  Operator=cos
  Trigonometric Function2 : Trigonometry  Operator=cos
  Unit Delay : UnitDelay  SampleTime=-1
  KsinwtExt : Outport
  KsinwtSin : Outport  Port=2
  KsinwtCos : Outport  Port=3
  Agm : Outport  Port=4
  Wm : Outport  Port=5
  wires:
  Trigonometric Function1/1 -> Gain/1
  Gain2/1 -> Trigonometric Function1/1
  Gain/1 -> Rslvr/1, KsinwtExt/1, Product/1, Product1/1
  Trigonometric Function/1 -> Product/2
  Trigonometric Function2/1 -> Product1/2
  Product1/1 -> Mux/2, KsinwtCos/1
  Gain1/1 -> Trigonometric Function/1, Trigonometric Function2/1
  Discrete Derivative/1 -> Wm/1
  RotorAgm/1 -> Discrete Derivative/1, Agm/1, Gain1/1
  Product/1 -> Mux/1, KsinwtSin/1
  Mux/1 -> Rslvr/2
  Constant/1 -> Add/1
  Add/1 -> Gain3/1, Unit Delay/1
  Unit Delay/1 -> Add/2
  Gain3/1 -> Gain2/1

== system PMSM_2017b_1013/Plant Dc Inverter Motor/Subsystem ==
  Fpwm : Inport
  Add : Sum
  Add2 : Sum  Inputs=+-
  Constant1 : Constant
  Constant2 : Constant  Value=Ts
  Constant3 : Constant  Value=Ts
  Divide : Product  Inputs=*/
  Gain : Gain  Gain=0.5
  Math Function : Math  Operator=reciprocal  SaturateOnIntegerOverflow=on
  Mod : Math  Operator=mod  SaturateOnIntegerOverflow=on
  Product : Product
  Relational Operator : RelationalOperator  Operator=<  OutDataTypeStr=boolean  RndMeth=Simplest
  Switch1 : Switch  Criteria=u2 > Threshold  Threshold=0.5
  Te4 : Scope
  Unit Delay : UnitDelay  InitialCondition=-1  SampleTime=-1
  Out1 : Outport
  wires:
  Constant2/1 -> Divide/2
  Relational Operator/1 -> Switch1/2
  Gain/1 -> Relational Operator/2
  Unit Delay/1 -> Add/2
  Constant1/1 -> Add/1
  Fpwm/1 -> Math Function/1
  Switch1/1 -> Product/2, Te4/1
  Math Function/1 -> Divide/1
  Add/1 -> Unit Delay/1, Mod/1
  Divide/1 -> Gain/1, Mod/2, Add2/1
  Mod/1 -> Add2/2, Switch1/1, Relational Operator/1
  Add2/1 -> Switch1/3
  Product/1 -> Out1/1
  Constant3/1 -> Product/1

== system PMSM_2017b_1013/SW/ADC ==
  note: 实际DSP程序中，在此模块中进行 电流/电压/旋变的采样信号的标定 ，
      |
      | 默认是仿真模式
  IabcSim : Inport
  RsvlrSinSim : Inport  Port=2
  RsvlrCosSim : Inport  Port=3
  Constant{,1..3} (4 alike) : Constant  Value=SimMode
  IabcRaw : Constant
  RsvlrCosRaw : Constant
  RsvlrSinRaw : Constant
  Switch{,1..3} (4 alike) : Switch  Criteria=u2 > Threshold  Threshold=0.5
      settings: AttributesFormatString=%<Criteria>
  UdcRaw : Constant
  UdcSim : Constant  Value=Udc
  Udc : Outport
  Iabc : Outport  Port=2
  RslvrSin : Outport  Port=3
  RslvrCos : Outport  Port=4
  wires:
  Constant/1 -> Switch/2
  UdcSim/1 -> Switch/1
  UdcRaw/1 -> Switch/3
  Switch/1 -> Udc/1
  IabcSim/1 -> Switch1/1
  IabcRaw/1 -> Switch1/3
  Constant1/1 -> Switch1/2
  Switch1/1 -> Iabc/1
  Switch2/1 -> RslvrSin/1
  Constant2/1 -> Switch2/2
  Constant3/1 -> Switch3/2
  RsvlrSinSim/1 -> Switch2/1
  RsvlrSinRaw/1 -> Switch2/3
  RsvlrCosRaw/1 -> Switch3/3
  Switch3/1 -> RslvrCos/1
  RsvlrCosSim/1 -> Switch3/1

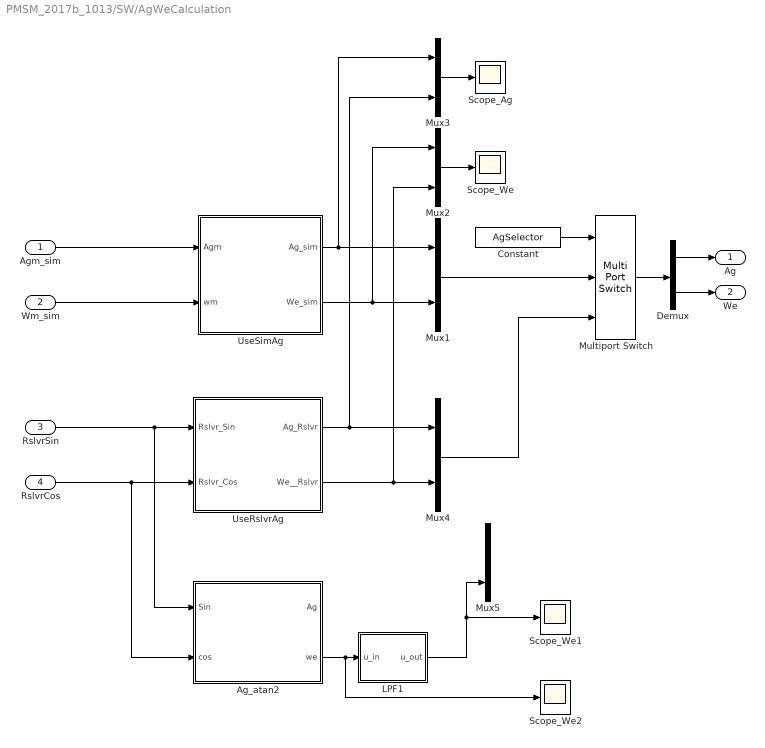
== system PMSM_2017b_1013/SW/AgWeCalculation ==
  Agm_sim : Inport
  Wm_sim : Inport  Port=2
  RslvrSin : Inport  Port=3
  RslvrCos : Inport  Port=4
  Ag_atan2 : Subsystem
  Constant : Constant  Value=AgSelector
  Demux : Demux  Outputs=2
  LPF1 : Subsystem
  Multiport Switch : MultiPortSwitch  DataPortOrder=Zero-based contiguous  Inputs=2
  Mux{1..5} (5 alike) : Mux  Inputs=2
  Scope_Ag : Scope
  Scope_We : Scope
  Scope_We1 : Scope
  Scope_We2 : Scope
  UseRslvrAg : Subsystem
  UseSimAg : Subsystem
  Ag : Outport
  We : Outport  Port=2
  wires:
  RslvrSin/1 -> Ag_atan2/1(Sin), UseRslvrAg/1(Rslvr_Sin)
  RslvrCos/1 -> Ag_atan2/2(cos), UseRslvrAg/2(Rslvr_Cos)
  Wm_sim/1 -> UseSimAg/2(wm)
  Agm_sim/1 -> UseSimAg/1(Agm)
  UseRslvrAg/1(Ag_Rslvr) -> Mux3/2, Mux4/1
  UseRslvrAg/2(We__Rslvr) -> Mux2/2, Mux4/2
  Mux1/1 -> Multiport Switch/2
  Constant/1 -> Multiport Switch/1
  Mux4/1 -> Multiport Switch/3
  Demux/1 -> Ag/1
  Demux/2 -> We/1
  UseSimAg/2(We_sim) -> Mux2/1, Mux1/2
  UseSimAg/1(Ag_sim) -> Mux3/1, Mux1/1
  Multiport Switch/1 -> Demux/1
  Mux3/1 -> Scope_Ag/1
  Mux2/1 -> Scope_We/1
  Ag_atan2/2(we) -> Scope_We2/1, LPF1/1(u_in)
  LPF1/1(u_out) -> Scope_We1/1, Mux5/2

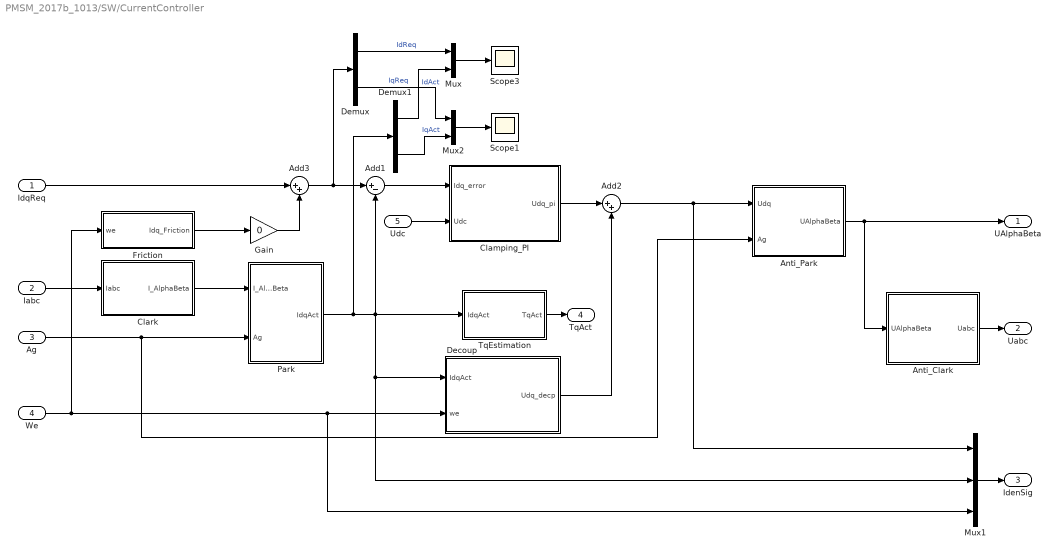
== system PMSM_2017b_1013/SW/CurrentController ==
  IdqReq : Inport
  Iabc : Inport  Port=2
  Ag : Inport  Port=3
  We : Inport  Port=4
  Udc : Inport  Port=5
  Add1 : Sum  Inputs=|+-
  Add2 : Sum  Inputs=|++
  Add3 : Sum  Inputs=|++
  Anti_Clark : Subsystem
  Anti_Park : Subsystem
  Clamping_PI : Subsystem
  Clark : Subsystem
  Decoup : Subsystem
  Demux : Demux  Outputs=2
  Demux1 : Demux  Outputs=2
  Friction : Subsystem
  Gain : Gain  Gain=0
  Mux : Mux  Inputs=2
  Mux1 : Mux  Inputs=3
  Mux2 : Mux  Inputs=2
  Park : Subsystem
  Scope1 : Scope
  Scope3 : Scope
  TqEstimation : Subsystem
  UAlphaBeta : Outport
  Uabc : Outport  Port=2
  IdenSig : Outport  Port=3
  TqAct : Outport  Port=4
  wires:
  We/1 -> Friction/1(we), Mux1/3, Decoup/2(we)
  Clark/1(I_AlphaBeta) -> Park/1(I_AlphaBeta)
  Iabc/1 -> Clark/1(Iabc)
  Ag/1 -> Anti_Park/2(Ag), Park/2(Ag)
  Anti_Park/1(UAlphaBeta) -> Anti_Clark/1(UAlphaBeta), UAlphaBeta/1
  Add1/1 -> Clamping_PI/1(Idq_error)
  Clamping_PI/1(Udq_pi) -> Add2/1
  Decoup/1(Udq_decp) -> Add2/2
  Udc/1 -> Clamping_PI/2(Udc)
  Anti_Clark/1(Uabc) -> Uabc/1
  Add2/1 -> Mux1/1, Anti_Park/1(Udq)
  Mux1/1 -> IdenSig/1
  Friction/1(Idq_Friction) -> Gain/1
  IdqReq/1 -> Add3/1
  Add3/1 -> Demux/1, Add1/1
  Gain/1 -> Add3/2
  Park/1(IdqAct) -> Demux1/1, TqEstimation/1(IdqAct), Mux1/2, Decoup/1(IdqAct), Add1/2
  Demux/1 -> Mux/1  "IdReq"
  Demux1/1 -> Mux/2  "IdAct"
  Mux2/1 -> Scope1/1
  Mux/1 -> Scope3/1
  Demux/2 -> Mux2/1  "IqReq"
  Demux1/2 -> Mux2/2  "IqAct"
  TqEstimation/1(TqAct) -> TqAct/1

== system PMSM_2017b_1013/SW/FpwmCalculation ==
  TqAct : Inport
  2-D Lookup Table : Lookup_n-D  NumberOfTableDimensions=1  BreakpointsForDimension1="[1  2  3  4]"  BreakpointsForDimension2=[1:3]  Table=[4000 6000 8000 10000]  InterpMethod=Flat  ExtrapMethod=Clip  InternalRulePriority=Speed  RndMeth=Simplest  InputSameDT=on
  Constant : Constant
  Constant1 : Constant  Value=10000
  Scope2 : Scope
  Switch : Switch  Criteria=u2 > Threshold  Threshold=0.5
  Fpwm : Outport
  wires:
  2-D Lookup Table/1 -> Switch/1
  TqAct/1 -> 2-D Lookup Table/1
  Switch/1 -> Scope2/1, Fpwm/1
  Constant/1 -> Switch/2
  Constant1/1 -> Switch/3

== system PMSM_2017b_1013/SW/SVPWM ==
  UAlphaBeta : Inport
  Udc : Inport  Port=2
  Fpwm : Inport  Port=3
  Demux : Demux  Outputs=2
  Math Function : Math  Operator=reciprocal  SaturateOnIntegerOverflow=on
  Sector Caculate : Subsystem
  T1T1 Caculate : Subsystem
  Tcm Caculate : Subsystem
  XYZ Caculate : Subsystem
  Tcm123 : Outport
  wires:
  Demux/2 -> Sector Caculate/2(Ubeta), XYZ Caculate/2(Ubeta)
  T1T1 Caculate/1(T1) -> Tcm Caculate/2(T1)
  Demux/1 -> Sector Caculate/1(Ualpha), XYZ Caculate/1(Ualpha)
  T1T1 Caculate/2(T2) -> Tcm Caculate/3(T2)
  Sector Caculate/1("N ") -> Tcm Caculate/1(N), T1T1 Caculate/1(N)
  XYZ Caculate/1(XYZ) -> T1T1 Caculate/2(XYZ)
  Math Function/1 -> XYZ Caculate/3(Tpwm), Tcm Caculate/4(Tpwm), T1T1 Caculate/3(Tpwm)
  Udc/1 -> XYZ Caculate/4(Udc)
  Tcm Caculate/1(Tcm1 Tcm2 Tcm3) -> Tcm123/1
  UAlphaBeta/1 -> Demux/1
  Fpwm/1 -> Math Function/1

== system PMSM_2017b_1013/SW/SpdController ==
  SpdReq : Inport
  We : Inport  Port=2
  Abs : Abs
  Add : Sum
  Add3 : Sum  Inputs=|+-
  Clamping_PI : Subsystem
  Clamping_PI1 : Subsystem  Commented=on
  Constant : Constant
  Discrete-Time Integrator : DiscreteIntegrator  SampleTime=-1  UpperSaturationLimit=UpperLimit  LowerSaturationLimit=LowerLimit  ICPrevOutput=DiscIntNeverNeededParam  ICPrevScaledInput=DiscIntNeverNeededParam
  EOT : Subsystem
  Gain : Gain  Gain=Tpwm
  Mux5 : Mux  Inputs=2
  Product : Product
  Scope1 : Scope
  Scope2 : Scope
  Scope3 : Scope
  Unit Delay : UnitDelay  SampleTime=-1
  we2wm : Gain  Gain=1/P
  wm2Nr : Gain  Gain=30/pi
  IdqReq : Outport
  wires:
  Mux5/1 -> Scope1/1
  we2wm/1 -> wm2Nr/1
  wm2Nr/1 -> Clamping_PI/2(SpdAct), Add3/2, Mux5/2  "SpdAct"
  EOT/1(IdqReq) -> IdqReq/1
  SpdReq/1 -> Mux5/1, Add3/1
  We/1 -> we2wm/1
  Add3/1 -> Abs/1, Clamping_PI1/1(Spd_error), Clamping_PI/1(Spd_error)
  Clamping_PI1/1(IqReq) -> Scope2/1
  Abs/1 -> Product/1
  Constant/1 -> Add/1
  Add/1 -> Gain/1, Unit Delay/1
  Unit Delay/1 -> Add/2
  Gain/1 -> Product/2
  Product/1 -> Discrete-Time Integrator/1
  Discrete-Time Integrator/1 -> Scope3/1  "ITAE"
  Clamping_PI/1(IqReq) -> EOT/1(IqReq)

== system PMSM_2017b_1013/SW/TqController ==
  note: Id=0控制
  TqReq : Inport
  IdReq : Constant  Value=0
  Mux : Mux  Inputs=2
  Nm->Iq : Gain  Gain=sqrt(2)/Kt
  IdqReq : Outport
  wires:
  IdReq/1 -> Mux/1
  Nm->Iq/1 -> Mux/2  "IqReq"
  Mux/1 -> IdqReq/1
  TqReq/1 -> Nm->Iq/1

== system PMSM_2017b_1013/Development Lib/UseMRASAg/MRAS ==
  ud : Inport
  uq : Inport  Port=2
  id : Inport  Port=3
  iq : Inport  Port=4
  Gain3 : Gain  Gain=15/2/pi
  Integrator : Integrator
  Subsystem : Subsystem
  Subsystem1 : Subsystem
  change theta : Subsystem
  w_e : Outport
  theta : Outport  Port=2
  wires:
  ud/1 -> Subsystem/1(ud)
  uq/1 -> Subsystem/2(uq)
  Subsystem/1(i_d) -> Subsystem1/3(i_d1)
  Subsystem/2(i_q) -> Subsystem1/4(i_q1)
  id/1 -> Subsystem1/1(id)
  iq/1 -> Subsystem1/2(iq)
  Subsystem1/1(w_e) -> Subsystem/3(we), Gain3/1, Integrator/1
  Gain3/1 -> w_e/1
  Integrator/1 -> change theta/1(In1)
  change theta/1(Out1) -> theta/1

== system PMSM_2017b_1013/Development Lib/UseSMOAg/Atan ==
  E_AlphaBeta : Inport
  Add : Sum
  Constant : Constant  Value=20000
  Fcn : Fcn  Expr=sqrt(u(1)^2+u(2)^2)
  Fcn1 : Fcn  Expr=atan(u(1)/u(2))
  Fcn2 : Fcn  Expr=-atan(u(1)/u(2))
  Gain : Gain  Gain=1/flux
  Mux : Mux  Inputs=2
  Ag_SMO : Outport
  we_SMO : Outport  Port=2
  wires:
  Fcn/1 -> Gain/1
  E_AlphaBeta/1 -> Fcn2/1, Fcn/1
  Gain/1 -> we_SMO/1, Mux/1
  Constant/1 -> Mux/2
  Mux/1 -> Fcn1/1
  Fcn1/1 -> Add/1
  Fcn2/1 -> Add/2
  Add/1 -> Ag_SMO/1  "e"

== system PMSM_2017b_1013/Development Lib/UseSMOAg/PLL  ==
  E_AlphaBeta : Inport
  Add : Sum  Inputs=+-
  Constant2 : Constant  Value=2*pi
  Demux : Demux  Outputs=2
  Discrete-Time Integrator2 : DiscreteIntegrator  SampleTime=-1  ICPrevOutput=DiscIntNeverNeededParam  ICPrevScaledInput=DiscIntNeverNeededParam
  Gain : Gain  Gain=-1
  LPF : Subsystem
  Mod : Math  Operator=mod  SaturateOnIntegerOverflow=on
  Product : Product
  Product1 : Product
  Scope : Scope  NumInputPorts=2
  Sin : Trigonometry
  Sin1 : Trigonometry  Operator=cos
  Subsystem : Subsystem
  Unit Delay : UnitDelay  SampleTime=-1
  Ag_SMO : Outport
  we_SMO : Outport  Port=2
  wires:
  Product1/1 -> Add/2
  Sin/1 -> Product1/2
  Product/1 -> Add/1
  Discrete-Time Integrator2/1 -> Unit Delay/1
  Add/1 -> Subsystem/1(e)  "e"
  Subsystem/1(Out1) -> Scope/1, LPF/1(u_in), Discrete-Time Integrator2/1
  Sin1/1 -> Product/1
  Gain/1 -> Product/2
  LPF/1(u_out) -> Scope/2, we_SMO/1
  Demux/1 -> Gain/1
  Demux/2 -> Product1/1
  E_AlphaBeta/1 -> Demux/1
  Unit Delay/1 -> Mod/1, Sin/1, Sin1/1
  Mod/1 -> Ag_SMO/1
  Constant2/1 -> Mod/2

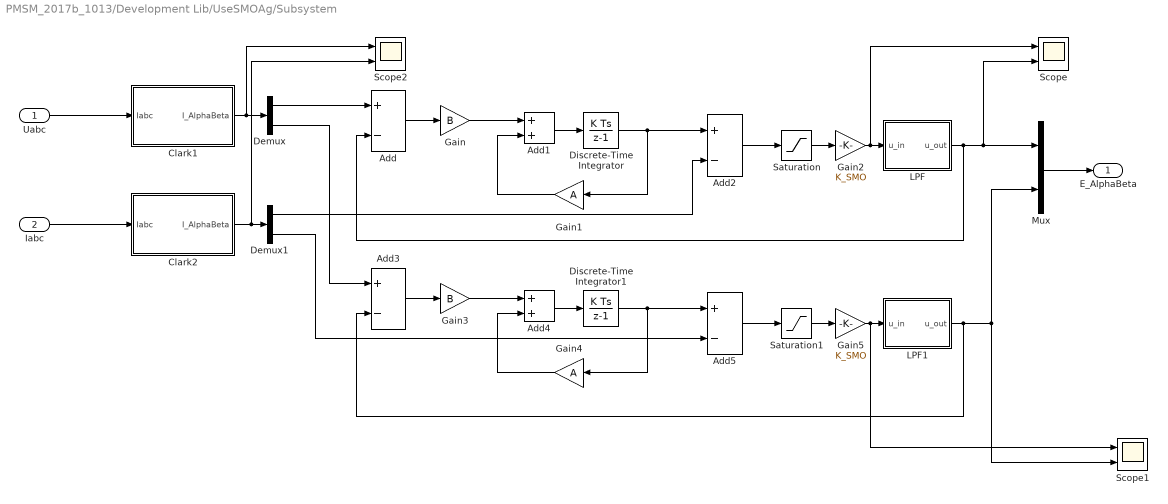
== system PMSM_2017b_1013/Development Lib/UseSMOAg/Subsystem ==
  Uabc : Inport
  Iabc : Inport  Port=2
  Add{,2..3,5} (4 alike) : Sum  Inputs=+-
  Add1 : Sum
  Add4 : Sum
  Clark1 : Subsystem
  Clark2 : Subsystem
  Demux : Demux  Outputs=2
  Demux1 : Demux  Outputs=2
  Discrete-Time Integrator : DiscreteIntegrator  InitialConditionSetting=State (most efficient)  SampleTime=-1  ICPrevOutput=DiscIntNeverNeededParam  ICPrevScaledInput=DiscIntNeverNeededParam
  Discrete-Time Integrator1 : DiscreteIntegrator  InitialConditionSetting=State (most efficient)  SampleTime=-1  ICPrevOutput=DiscIntNeverNeededParam  ICPrevScaledInput=DiscIntNeverNeededParam
  Gain : Gain  Gain=B
  Gain1 : Gain  Gain=A
  Gain2 : Gain  Gain=K_SMO
  Gain3 : Gain  Gain=B
  Gain4 : Gain  Gain=A
  Gain5 : Gain  Gain=K_SMO
  LPF : Subsystem
  LPF1 : Subsystem
  Mux : Mux  Inputs=2
  Saturation : Saturate  UpperLimit=1  LowerLimit=-1
  Saturation1 : Saturate  UpperLimit=1  LowerLimit=-1
  Scope : Scope  NumInputPorts=2
  Scope1 : Scope  NumInputPorts=2
  Scope2 : Scope  NumInputPorts=2
  E_AlphaBeta : Outport
  wires:
  Discrete-Time Integrator/1 -> Add2/1, Gain1/1
  Iabc/1 -> Clark2/1(Iabc)
  Demux1/1 -> Add2/2
  Uabc/1 -> Clark1/1(Iabc)
  Add2/1 -> Saturation/1
  Gain1/1 -> Add1/2
  Clark2/1(I_AlphaBeta) -> Scope2/2, Demux1/1
  Clark1/1(I_AlphaBeta) -> Scope2/1, Demux/1
  Add1/1 -> Discrete-Time Integrator/1
  Demux/1 -> Add/1
  Gain3/1 -> Add4/1
  Saturation1/1 -> Gain5/1
  Add/1 -> Gain/1
  Add3/1 -> Gain3/1
  Gain4/1 -> Add4/2
  Demux1/2 -> Add5/2
  Discrete-Time Integrator1/1 -> Gain4/1, Add5/1
  Add5/1 -> Saturation1/1
  Demux/2 -> Add3/1
  Gain5/1 -> Scope1/1, LPF1/1(u_in)
  LPF1/1(u_out) -> Mux/2, Scope1/2, Add3/2
  Add4/1 -> Discrete-Time Integrator1/1
  Gain/1 -> Add1/1
  Saturation/1 -> Gain2/1
  LPF/1(u_out) -> Mux/1, Scope/2, Add/2
  Gain2/1 -> Scope/1, LPF/1(u_in)
  Mux/1 -> E_AlphaBeta/1

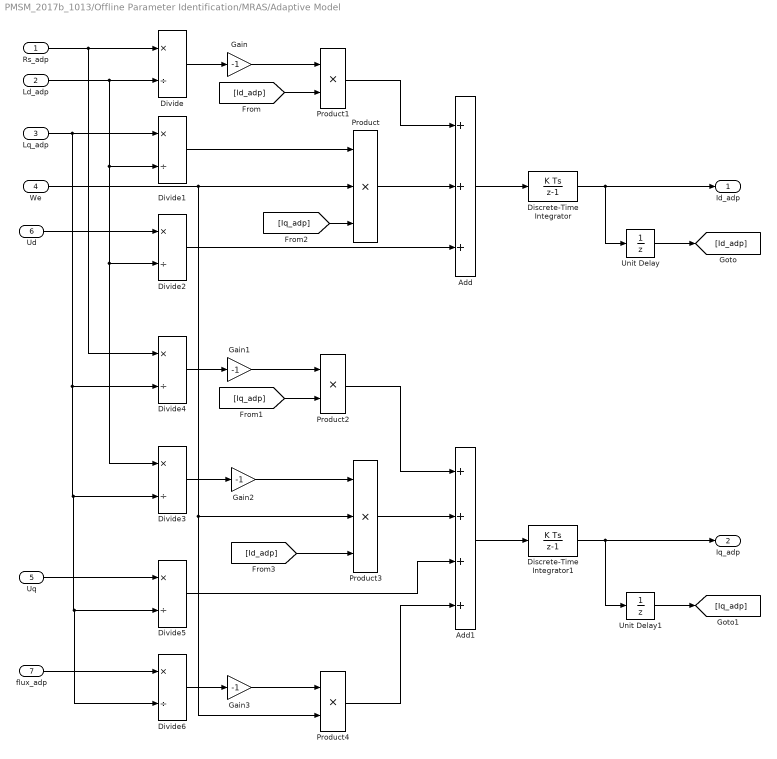
== system PMSM_2017b_1013/Offline Parameter Identification/MRAS/Adaptive Model ==
  Rs_adp : Inport
  Ld_adp : Inport  Port=2
  Lq_adp : Inport  Port=3
  We : Inport  Port=4
  Uq : Inport  Port=5
  Ud : Inport  Port=6
  flux_adp : Inport  Port=7
  Add : Sum  Inputs=3
  Add1 : Sum  Inputs=4
  Discrete-Time Integrator : DiscreteIntegrator  SampleTime=-1  UpperSaturationLimit=UpperLimit  LowerSaturationLimit=LowerLimit  ICPrevOutput=DiscIntNeverNeededParam  ICPrevScaledInput=DiscIntNeverNeededParam
  Discrete-Time Integrator1 : DiscreteIntegrator  SampleTime=-1  UpperSaturationLimit=UpperLimit  LowerSaturationLimit=LowerLimit  ICPrevOutput=DiscIntNeverNeededParam  ICPrevScaledInput=DiscIntNeverNeededParam
  Divide{,1..6} (7 alike) : Product  Inputs=*/
  Gain{,1..3} (4 alike) : Gain  Gain=-1
  Product : Product  Inputs=3
  Product1 : Product
  Product2 : Product
  Product3 : Product  Inputs=3
  Product4 : Product
  Unit Delay : UnitDelay  SampleTime=-1
  Unit Delay1 : UnitDelay  SampleTime=-1
  Id_adp : Outport
  Iq_adp : Outport  Port=2
  wires:
  Discrete-Time Integrator/1 -> Unit Delay/1, Id_adp/1
  Discrete-Time Integrator1/1 -> Unit Delay1/1, Iq_adp/1
  Add/1 -> Discrete-Time Integrator/1
  Rs_adp/1 -> Divide4/1, Divide/1
  Ld_adp/1 -> Divide2/2, Divide3/1, Divide1/2, Divide/2
  Divide/1 -> Gain/1
  Lq_adp/1 -> Divide4/2, Divide6/2, Divide5/2, Divide3/2, Divide1/1
  Ud/1 -> Divide2/1
  Divide1/1 -> Product/1
  Gain/1 -> Product1/1
  Product1/1 -> Add/1
  Product/1 -> Add/2
  Divide2/1 -> Add/3
  [Id_adp] -> Product1/2
  [Iq_adp] -> Product2/2
  Product2/1 -> Add1/1
  Gain1/1 -> Product2/1
  Divide4/1 -> Gain1/1
  Add1/1 -> Discrete-Time Integrator1/1
  [Iq_adp] -> Product/3
  Divide3/1 -> Gain2/1
  Gain2/1 -> Product3/1
  [Id_adp] -> Product3/3
  Product3/1 -> Add1/2
  Uq/1 -> Divide5/1
  Divide5/1 -> Add1/3
  flux_adp/1 -> Divide6/1
  Gain3/1 -> Product4/1
  Product4/1 -> Add1/4
  We/1 -> Product4/2, Product3/2, Product/2
  Divide6/1 -> Gain3/1
  Unit Delay/1 -> [Id_adp]
  Unit Delay1/1 -> [Iq_adp]

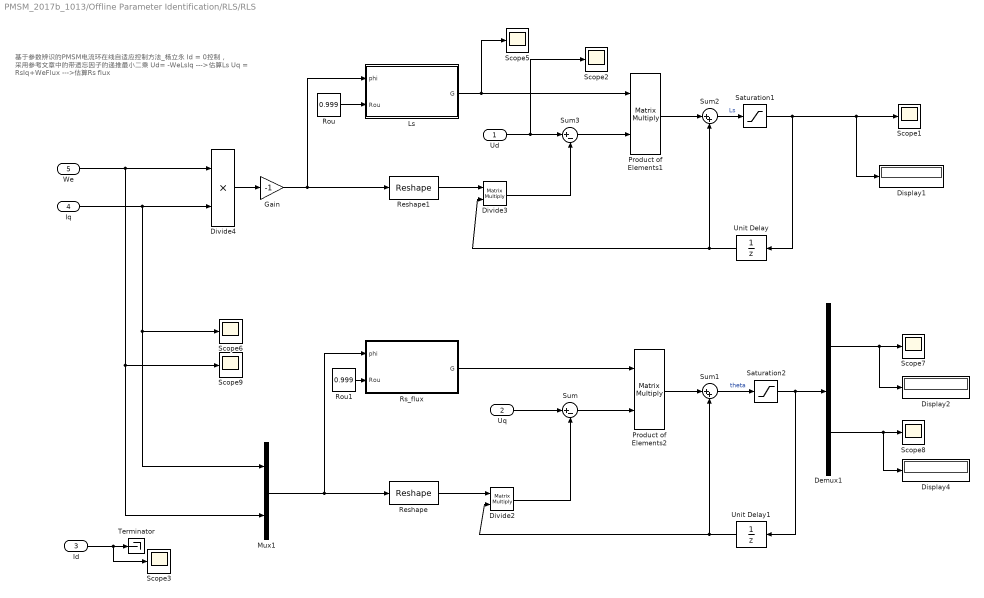
== system PMSM_2017b_1013/Offline Parameter Identification/RLS/RLS ==
  note: 基于参数辨识的PMSM电流环在线自适应控制方法_杨立永
      |
      | Id = 0控制， 采用参考文章中的带遗忘因子的递推最小二乘
      | Ud= -WeLsIq    --->估算Ls
      | Uq = RsIq+WeFlux   --->估算Rs flux
  Ud : Inport
  Uq : Inport  Port=2
  Id : Inport  Port=3
  Iq : Inport  Port=4
  We : Inport  Port=5
  Demux1 : Demux  Outputs=2
  Display1 : Display
  Display2 : Display
  Display4 : Display
  Divide2 : Product  Inputs=**  Multiplication=Matrix(*)
  Divide3 : Product  Inputs=**  Multiplication=Matrix(*)
  Divide4 : Product  Inputs=**
  Gain : Gain  Gain=-1
  Ls : Subsystem
  Mux1 : Mux  Inputs=2
  Product of Elements1 : Product  Multiplication=Matrix(*)
  Product of Elements2 : Product  Multiplication=Matrix(*)
  Reshape : Reshape  OutputDimensionality=Customize  OutputDimensions=[1,2]
  Reshape1 : Reshape  OutputDimensionality=Customize
  Rou : Constant  Value=0.999
  Rou1 : Constant  Value=0.999
  Rs_flux : Subsystem
  Saturation1 : Saturate  UpperLimit=1  LowerLimit=0
  Saturation2 : Saturate  UpperLimit=20  LowerLimit=0
  Scope{1..3,5..9} (8 alike) : Scope
  Sum : Sum  Inputs=|+-
  Sum1 : Sum  Inputs=|++
  Sum2 : Sum  Inputs=|++
  Sum3 : Sum  Inputs=|+-
  Terminator : Terminator
  Unit Delay : UnitDelay  InitialCondition=0.01  SampleTime=-1
  Unit Delay1 : UnitDelay  InitialCondition=[0.01;0.01]  SampleTime=-1
  wires:
  Demux1/2 -> Display4/1, Scope8/1
  Unit Delay1/1 -> Divide2/2, Sum1/2
  Divide2/1 -> Sum/2
  Mux1/1 -> Rs_flux/1(phi), Reshape/1
  Reshape/1 -> Divide2/1
  We/1 -> Scope9/1, Mux1/2, Divide4/1
  Product of Elements2/1 -> Sum1/1
  Iq/1 -> Scope6/1, Mux1/1, Divide4/2
  Sum1/1 -> Saturation2/1  "theta"
  Demux1/1 -> Display2/1, Scope7/1
  Divide4/1 -> Gain/1
  Product of Elements1/1 -> Sum2/1
  Unit Delay/1 -> Divide3/2, Sum2/2
  Reshape1/1 -> Divide3/1
  Ud/1 -> Scope2/1, Sum3/1
  Divide3/1 -> Sum3/2
  Sum3/1 -> Product of Elements1/2
  Ls/1(G) -> Scope5/1, Product of Elements1/1
  Sum2/1 -> Saturation1/1  "Ls"
  Rou/1 -> Ls/2(Rou)
  Sum/1 -> Product of Elements2/2
  Rs_flux/1(G) -> Product of Elements2/1
  Gain/1 -> Ls/1(phi), Reshape1/1
  Uq/1 -> Sum/1
  Id/1 -> Scope3/1, Terminator/1
  Saturation2/1 -> Unit Delay1/1, Demux1/1
  Saturation1/1 -> Unit Delay/1, Display1/1, Scope1/1
  Rou1/1 -> Rs_flux/2(Rou)

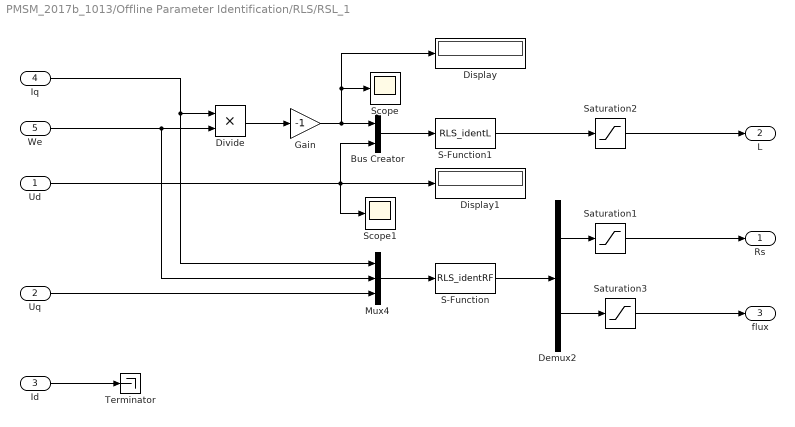
== system PMSM_2017b_1013/Offline Parameter Identification/RLS/RSL_1 ==
  Ud : Inport
  Uq : Inport  Port=2
  Id : Inport  Port=3
  Iq : Inport  Port=4
  We : Inport  Port=5
  Bus Creator : BusCreator  Inputs=2
  Demux2 : Demux  Outputs=2
  Display : Display
  Display1 : Display
  Divide : Product  Inputs=**
  Gain : Gain  Gain=-1
  Mux4 : Mux  Inputs=3
  S-Function : S-Function  FunctionName=RLS_identRF  SFunctionDeploymentMode=off  EnableBusSupport=off
  S-Function1 : S-Function  FunctionName=RLS_identL  SFunctionDeploymentMode=off  EnableBusSupport=off
  Saturation1 : Saturate  UpperLimit=30  LowerLimit=0
  Saturation2 : Saturate  UpperLimit=1  LowerLimit=0
  Saturation3 : Saturate  UpperLimit=1  LowerLimit=0
  Scope : Scope
  Scope1 : Scope
  Terminator : Terminator
  Rs : Outport
  L : Outport  Port=2
  flux : Outport  Port=3
  wires:
  Divide/1 -> Gain/1
  Gain/1 -> Display/1, Scope/1, Bus Creator/1
  Bus Creator/1 -> S-Function1/1
  S-Function1/1 -> Saturation2/1
  Mux4/1 -> S-Function/1
  S-Function/1 -> Demux2/1
  Demux2/1 -> Saturation1/1
  Iq/1 -> Divide/1, Mux4/1
  We/1 -> Divide/2, Mux4/2
  Ud/1 -> Bus Creator/2, Display1/1, Scope1/1
  Uq/1 -> Mux4/3
  Demux2/2 -> Saturation3/1
  Saturation2/1 -> L/1
  Saturation3/1 -> flux/1
  Id/1 -> Terminator/1
  Saturation1/1 -> Rs/1
